simulink model "simulink_test"  (R2022b)
settings: Solver=VariableStepAuto  StartTime=0.0  StopTime=2  RelTol=1e-3
undefined symbols (not defined in the file or in its folder): duration, effort, index, joint3, joint_name, model_name, open_manipulator
libraries: robotgazebolib x14
settings Model: Creator=marin  LastModifiedBy=marin

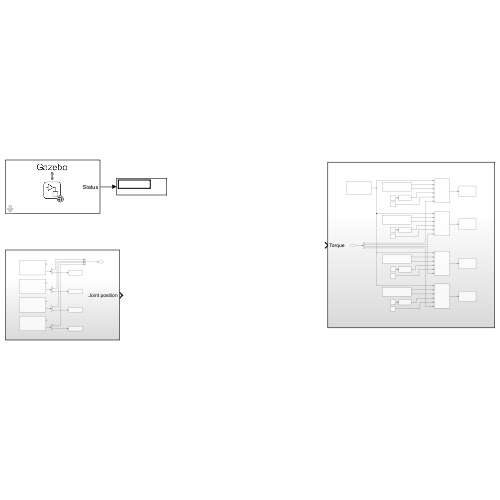
[thumbnail: Simulink's stored preview of the top-level diagram]
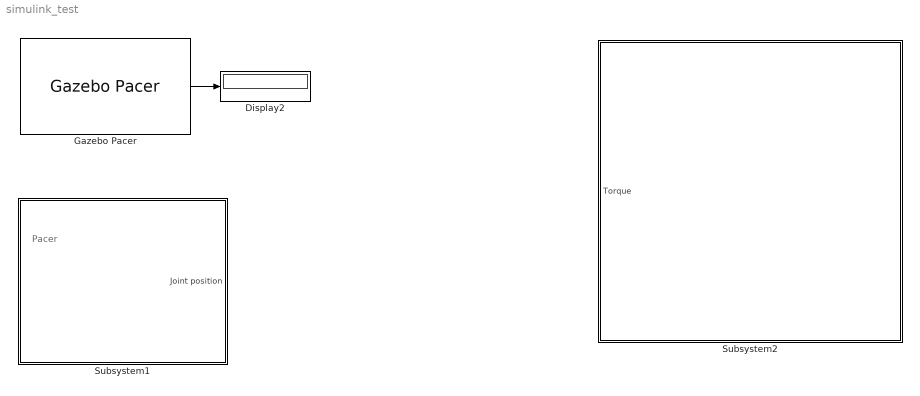
== system simulink_test ==
  note: Pacer
  Display2 : Display
  Gazebo Pacer : robotgazebolib/Gazebo Pacer  ResetBehavior=Reset Gazebo simulation time and scene  SampleTime=0.001
  Subsystem1 : Subsystem
  Subsystem2 : Subsystem
  wires:
  Gazebo Pacer/1 -> Display2/1

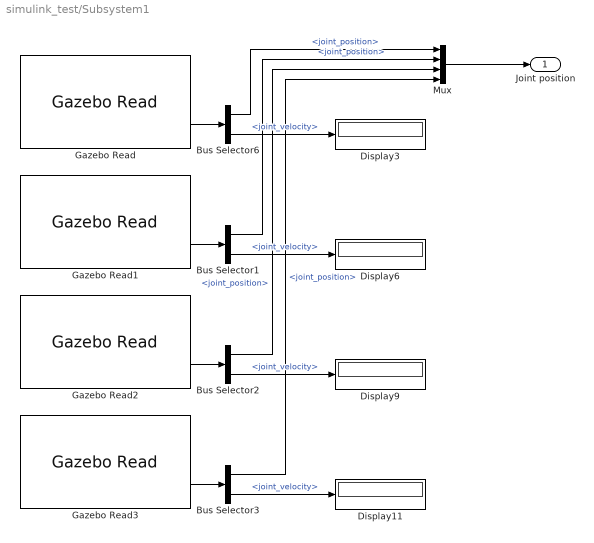
== system simulink_test/Subsystem1 ==
  Bus Selector{1..3,6} (4 alike) : BusSelector  OutputSignals=joint_position,joint_velocity
  Display{3,6,9,11} (4 alike) : Display
  Gazebo Read{,1..3} (4 alike) : robotgazebolib/Gazebo Read  topicSource=From Gazebo  topic=/gazebo/ground_truth/joint_state/open_manipulator/joint3  messageType=gazebo_msgs/JointState  sampleTime=0.001  fixedAxisBusStatus=off  jointAxisCount=2
  Mux : Mux
  Joint position : Outport
  wires:
  Bus Selector1/2 -> Display6/1  "<joint_velocity>"
  Gazebo Read/2 -> Bus Selector6/1
  Gazebo Read1/2 -> Bus Selector1/1
  Bus Selector6/2 -> Display3/1  "<joint_velocity>"
  Bus Selector2/2 -> Display9/1  "<joint_velocity>"
  Bus Selector2/1 -> Mux/3  "<joint_position>"
  Gazebo Read2/2 -> Bus Selector2/1
  Bus Selector1/1 -> Mux/2  "<joint_position>"
  Mux/1 -> Joint position/1
  Bus Selector3/2 -> Display11/1  "<joint_velocity>"
  Bus Selector3/1 -> Mux/4  "<joint_position>"
  Gazebo Read3/2 -> Bus Selector3/1
  Bus Selector6/1 -> Mux/1  "<joint_position>"

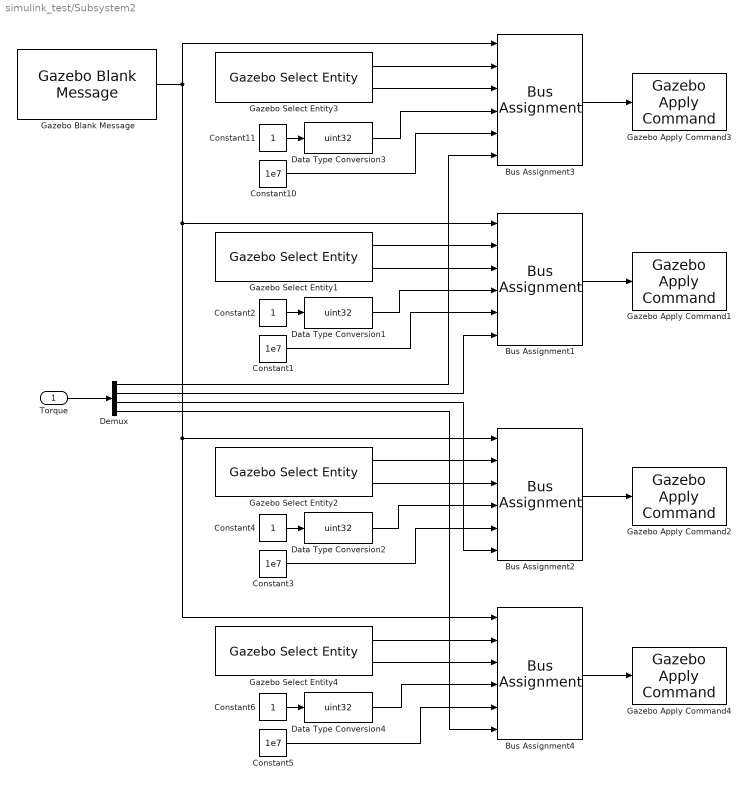
== system simulink_test/Subsystem2 ==
  Torque : Inport
  Bus Assignment{1..4} (4 alike) : BusAssignment  AssignedSignals=model_name,joint_name,index,duration.nano_seconds,effort
  Constant{1,3,5,10} (4 alike) : Constant  Value=1e7
  Constant{2,4,6,11} (4 alike) : Constant
  Data Type Conversion{1..4} (4 alike) : DataTypeConversion  OutDataTypeStr=uint32  SaturateOnIntegerOverflow=off  RndMeth=Floor
  Demux : Demux
  Gazebo Apply Command{1..4} (4 alike) : robotgazebolib/Gazebo Apply Command  cmdType=ApplyJointTorque  sampleTime=0.01
  Gazebo Blank Message : robotgazebolib/Gazebo Blank Message  msgType=ApplyJointTorque  sampleTime=0.01  busName='Gazebo_SL_Bus_gazebo_msgs_ApplyJointTorque'
  Gazebo Select Entity{1..4} (4 alike) : robotgazebolib/Gazebo Select Entity  modelElemName=open_manipulator/joint3  outputArraySize=128  OutputLabel=Joint  SelectType=Joint
  wires:
  Constant11/1 -> Data Type Conversion3/1
  Gazebo Select Entity3/1 -> Bus Assignment3/2
  Constant10/1 -> Bus Assignment3/5
  Gazebo Select Entity3/2 -> Bus Assignment3/3
  Bus Assignment3/1 -> Gazebo Apply Command3/1
  Data Type Conversion3/1 -> Bus Assignment3/4
  Torque/1 -> Demux/1
  Bus Assignment1/1 -> Gazebo Apply Command1/1
  Data Type Conversion1/1 -> Bus Assignment1/4
  Constant1/1 -> Bus Assignment1/5
  Gazebo Select Entity1/2 -> Bus Assignment1/3
  Constant2/1 -> Data Type Conversion1/1
  Bus Assignment2/1 -> Gazebo Apply Command2/1
  Data Type Conversion2/1 -> Bus Assignment2/4
  Constant3/1 -> Bus Assignment2/5
  Gazebo Select Entity2/2 -> Bus Assignment2/3
  Constant4/1 -> Data Type Conversion2/1
  Bus Assignment4/1 -> Gazebo Apply Command4/1
  Data Type Conversion4/1 -> Bus Assignment4/4
  Constant5/1 -> Bus Assignment4/5
  Gazebo Select Entity4/2 -> Bus Assignment4/3
  Constant6/1 -> Data Type Conversion4/1
  Gazebo Select Entity2/1 -> Bus Assignment2/2
  Gazebo Select Entity4/1 -> Bus Assignment4/2
  Gazebo Blank Message/1 -> Bus Assignment3/1, Bus Assignment4/1, Bus Assignment2/1, Bus Assignment1/1
  Demux/1 -> Bus Assignment3/6
  Demux/2 -> Bus Assignment1/6
  Demux/3 -> Bus Assignment2/6
  Demux/4 -> Bus Assignment4/6
  Gazebo Select Entity1/1 -> Bus Assignment1/2
